simulink model "simulink_model"  (R2022b)
settings: Solver=VariableStepAuto  StartTime=0.0  StopTime=5*N  RelTol=1e-3
libraries: cstblocks x1
settings Model: Creator=chuan  LastModifiedBy=chuan

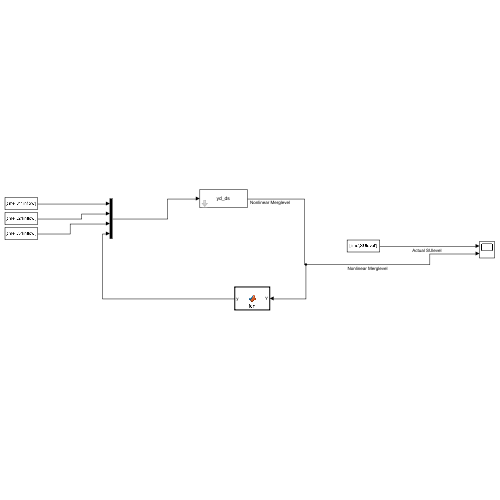
[thumbnail: Simulink's stored preview of the top-level diagram]
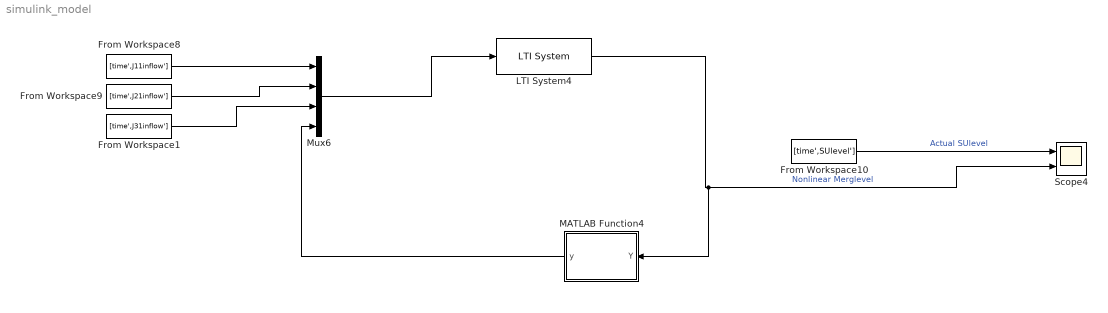
== system simulink_model ==
  From Workspace1 : FromWorkspace  VariableName=[time',J31inflow']
  From Workspace10 : FromWorkspace  VariableName=[time',SUlevel']
  From Workspace8 : FromWorkspace  VariableName=[time',J11inflow']
  From Workspace9 : FromWorkspace  VariableName=[time',J21inflow']
  LTI System4 : cstblocks/LTI System  sys=yd_ds  IC=[]
  MATLAB Function4 : MATLAB Function  TreatAsAtomicUnit=on
  Mux6 : Mux
  Scope4 : Scope  NumInputPorts=2
  wires:
  From Workspace9/1 -> Mux6/2
  From Workspace8/1 -> Mux6/1
  From Workspace10/1 -> Scope4/1  "Actual SUlevel"
  Mux6/1 -> LTI System4/1
  LTI System4/1 -> MATLAB Function4/1(Y), Scope4/2  "Nonlinear Merglevel"
  MATLAB Function4/1(y) -> Mux6/4
  From Workspace1/1 -> Mux6/3

== matlab function simulink_model/MATLAB Function4 ==
  data: Y input; y output
function y = fcn(Y)
Cd = 0.65;
A0 = 25;
g = 9.81;
Z0 = 0;
Yfull = 5;
H_star = Z0 + Yfull;

Y = max(Y,0);
H1 = Y + Z0;

if H1 >= H_star
    He = H1 - (Z0 + Yfull/2);
    y = Cd*A0*sqrt(2*g*He);
else
    CwL = (Cd*A0*sqrt(g))/(Yfull);
    y = CwL*(H1-Z0)^(1.5);
end
